simulink model "PV_Array"  (R2020a)
settings: Solver=VariableStepAuto  StartTime=0.0  StopTime=10.0  RelTol=1e-3
libraries: simulink x3, powerlib x2, re_lib x1
settings Model: Creator=royde  LastModifiedBy=royde

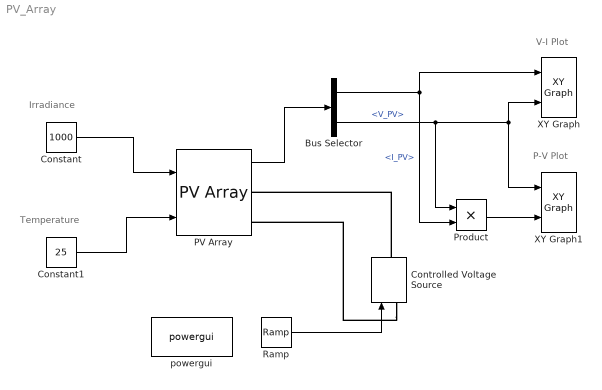
== system PV_Array ==
  note: Irradiance
  note: Temperature
  note: V-I Plot
  note: P-V Plot
  Bus Selector : BusSelector  OutputSignals=I_PV,V_PV
  Constant : Constant  Value=1000
  Constant1 : Constant  Value=25
  Controlled Voltage Source : powerlib/Electrical Sources/Controlled Voltage Source  Initialize=on  Source_Type=AC  Amplitude=0  Phase=0  Frequency=0  Measurements=None
  PV Array : re_lib/Solar/PV Array  Npar=1  Nser=1  PlotType=array @ 1000 W/m2 & specified temperatures  S_vec="[ 1000  500  100 ]"  Temp_C_vec="[ 45 25  ]"  ModuleName=SunPower SER-220P  PlotWhenSelected=off  Pm=219.9716  Ncell=60  Voc=36.3  Isc=8.3  Vm=29.02  Im=7.58  beta_Voc_pc=-0.35501  alpha_Isc_pc=0.043795  beta_Voc=-0.12887  alpha_Isc=0.003635  IL=8.3331  I0=2.2787e-10  nI=0.97003  Rsh=95.1262  Rs=0.37924  RobustModel=off  RobustCellTemperature=25  BAL=on  Tc=1e-6  Tfilter=5e-5
  Product : Product
  Ramp : simulink/Sources/Ramp  slope=5  start=0  InitialOutput=0
  XY Graph : simulink/Sinks/XY Graph  xmin=0  xmax=9  ymin=0  ymax=40  st=-1
  XY Graph1 : simulink/Sinks/XY Graph  xmin=0  xmax=40  ymin=0  ymax=250  st=-1
  powergui : powerlib/powergui  Priority=1  SimulationMode=Continuous  SampleTime=50e-6  frequency=60  Iterations=50  frequencyindice=0  Pbase=100e6  ErrMax=1e-4  UnitsV=kV  UnitsW=MW  buscounter=0  FunctionMessages=off  echomessages=off  EnableUseOfTLC=off  CurrentSourceSwitches=off  DisableSnubberDevices=off  DisableRonSwitches=off  DisableVfSwitches=off  DisplayEquations=off  AutomaticDiscreteSolvers=off  SolverType=Tustin/Backward Euler (TBE)  Interpol=off  ExternalGateDelay=off  methode=off  Ts=100  x0status=blocks  SPID=on  SwTol=0  HookPort=off  NonlinearTolerance=1e-4  nMaxIteration=100  ContinueOnMaxIteration=off  RestoreLinks=warning  ResistiveCurrentMeasurement=off  Frange=[0:2:500]  Ylog=off  Xlog=on  ShowGrid=off  save=off  variable=ZData  structure=0  ZoomFFT=off  StartTime=0.0  cycles=1  DisplayStyle=1  fundamental=60  FreqAxis=off  MaxFrequency=1000  frequencyindicesteady=1  RmsSteady=1  display=off
  wires:
  Constant/1 -> PV Array/1
  Constant1/1 -> PV Array/2
  PV Array/1 -> Bus Selector/1
  Ramp/1 -> Controlled Voltage Source/1
  Product/1 -> XY Graph1/2
  Bus Selector/1 -> Product/2, XY Graph/1  "<I_PV>"
  Bus Selector/2 -> Product/1, XY Graph1/1, XY Graph/2  "<V_PV>"
  connections:
  Controlled Voltage Source/RConn1 -- PV Array/RConn1
  Controlled Voltage Source/LConn1 -- PV Array/RConn2
